simulink model "MBD_Simple_Code_Generation"  (R2021b)
settings: Solver=FixedStepDiscrete  StartTime=0.0  StopTime=10.0  FixedStep=0.001  RelTol=1e-3
model workspace (MAT data in the model file):
  Noso = Simulink.Parameter
  Noso.Value = 3
  Noso.DataType = 'uint8'
  Noso.Min = 0
  Noso.Max = 5
  Noso.Complexity = 'real'
  Noso.Dimensions = [1 1]
  Param = Simulink.Parameter
  Param.DataType = 'auto'
  Param.Complexity = 'real'
  Param.Dimensions = [0 0]
  Param1 = Simulink.Parameter
  Param1.DataType = 'auto'
  Param1.Complexity = 'real'
  Param1.Dimensions = [0 0]
  Param2 = Simulink.Parameter
  Param2.DataType = 'auto'
  Param2.Complexity = 'real'
  Param2.Dimensions = [0 0]
  Param3 = Simulink.Parameter
  Param3.DataType = 'auto'
  Param3.Complexity = 'real'
  Param3.Dimensions = [0 0]
  Param4 = Simulink.Parameter
  Param4.DataType = 'auto'
  Param4.Complexity = 'real'
  Param4.Dimensions = [0 0]
settings Model: Creator=waleed.elshemy  LastModifiedBy=waleed.elshemy
settings OptimizationCC: DefaultParameterBehavior=Inlined  UseDivisionForNetSlopeComputation=on  GainParamInheritBuiltInType=on  UseFloatMulNetSlope=on  InlineInvariantSignals=on  PassReuseOutputArgsAs=Individual arguments  ZeroExternalMemoryAtStartup=off  ZeroInternalMemoryAtStartup=off  NoFixptDivByZeroProtection=on  EfficientFloat2IntCast=on  LifeSpan=1  OptimizeBlockOrder=speed  DifferentSizesBufferReuse=on  EfficientTunableParamExpr=on
settings DebuggingCC: ParameterTunabilityLossMsg=error
settings HardwareCC: ProdBitPerPointer=32  ProdBitPerSizeT=32  ProdBitPerPtrDiffT=32  ProdLargestAtomicFloat=None  ProdWordSize=32  ProdLongLongMode=on  ProdHWDeviceType=Atmel->AVR (32-bit)
settings SFSimCC: MATLABDynamicMemAlloc=off
settings RTWCC: Description=Embedded Coder  SystemTargetFile=ert.tlc  TemplateMakefile=ert_default_tmf
settings CodeAppCC: ForceParamTrailComments=on  IgnoreCustomStorageClasses=off  OperatorAnnotations=on  SimulinkDataObjDesc=on  SFDataObjDesc=on  CustomSymbolStrGlobalVar=rt$N$M  CustomSymbolStrType=$N$M  CustomSymbolStrFcn=$N$M$F  CustomSymbolStrMacro=$N$M  InsertBlockDesc=on
settings ERTTargetCC: TargetLangStandard=C99 (ISO)  GenerateSampleERTMain=on  IncludeMdlTerminateFcn=off  CombineSignalStateStructs=on  SuppressErrorStatus=on  SupportAbsoluteTime=off  SupportComplex=off  InlinedParameterPlacement=NonHierarchical  ERTCustomFileTemplate=example_file_process.tlc  ERTFilePackagingFormat=CompactWithDataFile

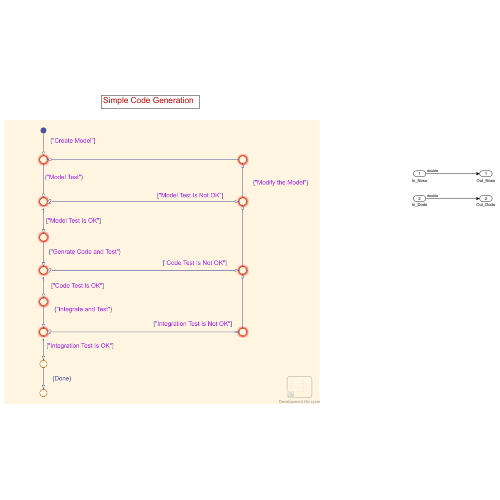
[thumbnail: Simulink's stored preview of the top-level diagram]
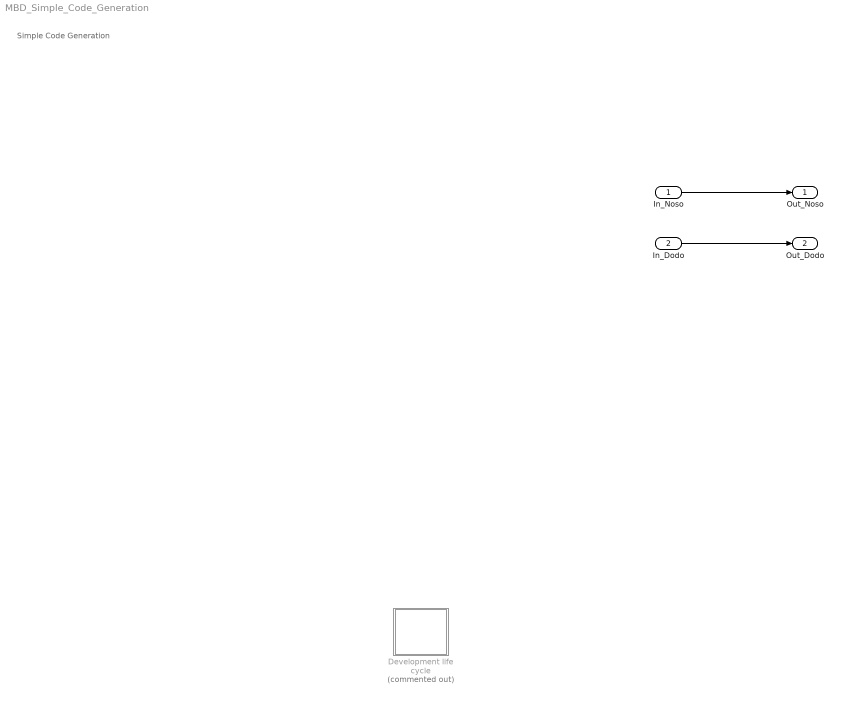
== system MBD_Simple_Code_Generation ==
  note: Simple Code Generation
  In_Noso : Inport
  In_Dodo : Inport  Port=2
  Development life cycle : Stateflow chart  Commented=on  TreatAsAtomicUnit=on
  Out_Noso : Outport
  Out_Dodo : Outport  Port=2
  wires:
  In_Noso/1 -> Out_Noso/1
  In_Dodo/1 -> Out_Dodo/1

== stateflow chart MBD_Simple_Code_Generation/Development life cycle ==
  (default) -> (junction 1) : ["Create Model"]
  (junction 10) -> (junction 1)
  (junction 1) -> (junction 3) : {"Model Test"}
  (junction 8) -> (junction 10) : {"Modify the Model"}
  (junction 3) -> (junction 8) [order 2] : ["Model Test Is Not OK"]
  (junction 3) -> (junction 5) [order 1] : ["Model Test Is OK"]
  (junction 17) -> (junction 8)
  (junction 5) -> (junction 13) : {"Genrate Code and Test"}
  (junction 13) -> (junction 17) [order 2] : ["Code Test Is Not OK"]
  (junction 13) -> (junction 15) [order 1] : ["Code Test Is OK"]
  (junction 24) -> (junction 17)
  (junction 15) -> (junction 20) : {"Integrate and Test"}
  (junction 20) -> (junction 24) [order 2] : ["Integration Test Is Not OK"]
  (junction 20) -> (junction 22) [order 1] : ["Integration Test Is OK"]
  (junction 22) -> (junction 27) : {Done}
